simulink model "prct_model_IMV"  (R2018a)
settings: Solver=FixedStepDiscrete  StartTime=0.0  StopTime=3.2  FixedStep=0.01  RelTol=1e-3
model workspace (MAT data in the model file):
  IMV_Time = Simulink.Signal
  IMV_Time.DataType = 'single'
  IMV_Time.Dimensions = -1
  IMV_Time.DimensionsMode = 'auto'
  IMV_Time.Complexity = 'auto'
  IMV_Time.SampleTime = -1
  IMV_Time.SamplingMode = 'auto'
values from neighbouring files (symbols this model uses):
  Diesel_Viscocity = 875.0    [HPP18_DD.sldd]
  Discharge_Coefficient = 0.7    [HPP18_DD.sldd]
  Divide_Constant = 4.0    [HPP18_DD.sldd]
  meterToliter = 1000.0    [HPP18_DD.sldd]
  Orifices_Dia = 0.0035    [HPP18_DD.sldd]
  Pressure_UnitConversion = 200000.0    [HPP18_DD.sldd]
  Time_ScalingFactor = 1000.0    [HPP18_DD.sldd]
undefined symbols (not defined in the file or in its folder): sigbuilder_block
libraries: simulink x2
settings Model: DataDictionary=Pract_IMV.sldd  Creator=Sohan  LastModifiedBy=Sohan
settings OptimizationCC: BlockReduction=off  DefaultParameterBehavior=Inlined  UseDivisionForNetSlopeComputation=on  EnhancedBackFolding=on  PassReuseOutputArgsAs=Individual arguments  EfficientFloat2IntCast=on  LifeSpan=inf  OptimizeBlockOrder=speed  DifferentSizesBufferReuse=on  OptimizationCustomize=off
settings DebuggingCC: SignalInfNanChecking=error  SignalRangeChecking=error  ReadBeforeWriteMsg=EnableAllAsError  WriteAfterWriteMsg=EnableAllAsError  WriteAfterReadMsg=EnableAllAsError  AlgebraicLoopMsg=error  ArtificialAlgebraicLoopMsg=error  SaveWithDisabledLinksMsg=error  SaveWithParameterizedLinksMsg=error  BlockPriorityViolationMsg=error  SolverPrmCheckMsg=error  InheritedTsInSrcMsg=error  SigSpecEnsureSampleTimeMsg=error  CheckMatrixSingularityMsg=error  IntegerOverflowMsg=error  ParameterUnderflowMsg=error  ParameterPrecisionLossMsg=error  ParameterTunabilityLossMsg=error  UnderSpecifiedDataTypeMsg=error  UnnecessaryDatatypeConvMsg=warning  VectorMatrixConversionMsg=error  SignalLabelMismatchMsg=error  UnconnectedInputMsg=error  UnconnectedOutputMsg=error  UnconnectedLineMsg=error  SFcnCompatibilityMsg=error  UniqueDataStoreMsg=warning  BusObjectLabelMismatch=error  RootOutportRequireBusObject=error  AssertControl=DisableAll  ModelReferenceIOMsg=error  ModelReferenceIOMismatchMessage=error  UnknownTsInhSupMsg=error  ModelReferenceDataLoggingMessage=error  StateNameClashWarn=warning  StrictBusMsg=ErrorOnBusTreatedAsVector  SFInvalidInputDataAccessInChartInitDiag=error  SFTransitionOutsideNaturalParentDiag=error  SFUnreachableExecutionPathDiag=error
settings SFSimCC: MATLABDynamicMemAlloc=off
settings RTWCC: SystemTargetFile=ert.tlc  TemplateMakefile=ert_default_tmf  GenerateReport=on  IncludeHyperlinkInReport=on  LaunchReport=on  GenerateTraceInfo=on  GenerateTraceReport=on  GenerateTraceReportSl=on  GenerateTraceReportSf=on  GenerateTraceReportEml=on
settings CodeAppCC: ForceParamTrailComments=on  IgnoreCustomStorageClasses=off  OperatorAnnotations=on  SimulinkDataObjDesc=on  SFDataObjDesc=on  MangleLength=4  InsertBlockDesc=on  ReqsInCode=on
settings ERTTargetCC: TargetLangStandard=C99 (ISO)  UtilityFuncGeneration=Shared location  GenerateSampleERTMain=on  IncludeMdlTerminateFcn=off  SuppressErrorStatus=on  SupportAbsoluteTime=off  SupportNonFinite=off  ParenthesesLevel=Maximum  CastingMode=Standards  GenerateSharedConstants=off  InlinedParameterPlacement=NonHierarchical  ERTCustomFileTemplate=example_file_process.tlc  PreserveExpressionOrder=on  PreserveIfCondition=on  EnableSignedLeftShifts=off  EnableSignedRightShifts=off
settings ConfigComp: CovEnable=on  RecordCoverage=on  CovMetricSettings=dcmwe  CovModelRefEnable=on  DVMaxProcessTime=333  DVModelCoverageObjectives=MCDC  DVTestSuiteOptimization=CombinedObjectives (Nonlinear Extended)  DVDetectDeadLogic=on  DVDetectFloatOverflow=off  DVSaveReport=on

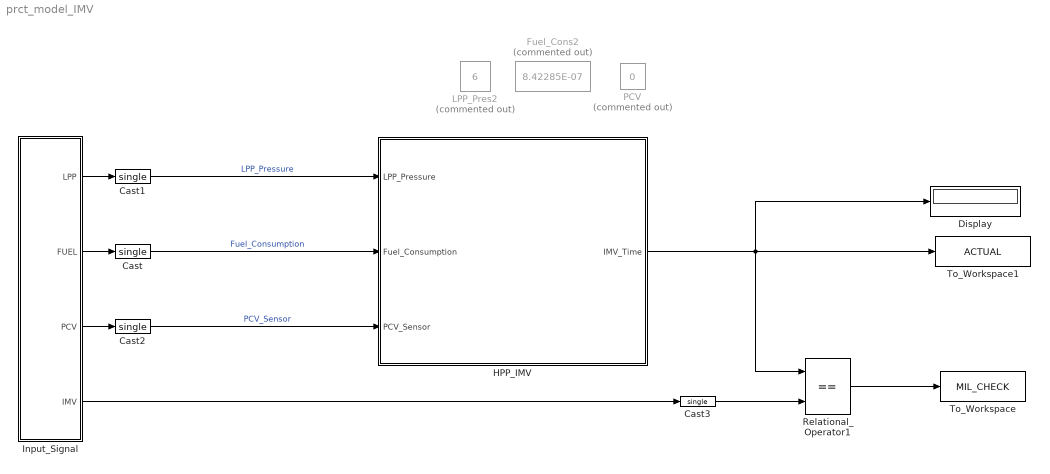
== system prct_model_IMV ==
  Cast{,1..3} (4 alike) : DataTypeConversion  OutDataTypeStr=single
  Display : Display
  Fuel_Cons2 : Constant  Commented=on  Value=8.42285E-07
  HPP_IMV : Subsystem  TreatAsAtomicUnit=on
  Input_Signal : Subsystem  Tag=STV Subsys  LoadFcn=sigbuilder_block('load');  StartFcn=sigbuilder_block('start');  StopFcn=sigbuilder_block('stop');  ClipboardFcn=sigbuilder_block('clipboard');  mask(Sigbuilder block){tuvar=[0:10]}
      mask help: Simulink:masks:SigbuilderBlock_MD
      mask init:
      | if ~strcmp(get_param(bdroot(gcbh),'SimulationStatus'),'stopped') tuvar = sigbuilder_block('maskInit'); end
      settings: CopyFcn=sigbuilder_block('copy');  DeleteFcn=sigbuilder_block('delete');  ModelCloseFcn=sigbuilder_block('modelClose');  PreSaveFcn=sigbuilder_block('preSave');  PauseFcn=sigbuilder_block('pause');  ContinueFcn=sigbuilder_block('continue');  NameChangeFcn=sigbuilder_block('namechange');  OpenFcn=sigbuilder_block('open',[433.2 159.6 550.8 400.2 ]);  CloseFcn=sigbuilder_block('close');
      mask Display: plot(0, 0, 100, 100,[2, 2, 32, 32, 2], [68, 8, 8, 68, 68],[32, 2], [38, 38], [32, 19, 2],[53, 60, 44], [32, 17, 17, 2],[16, 16, 31, 31]);txt = getActiveGroup(gcbh);text(2, 100, txt,'verticalAlignment', 'top');
  LPP_Pres2 : Constant  Commented=on  Value=6  OutDataTypeStr=single
  PCV : Constant  Commented=on  Value=0  OutDataTypeStr=single
  Relational_Operator1 : RelationalOperator  Operator===  OutDataTypeStr=boolean
  To_Workspace : ToWorkspace  VariableName=MIL_CHECK  SaveFormat=Timeseries  SampleTime=-1
  To_Workspace1 : ToWorkspace  VariableName=ACTUAL  SaveFormat=Timeseries  SampleTime=-1
  wires:
  Input_Signal/1(LPP) -> Cast1/1
  Relational_Operator1/1 -> To_Workspace/1
  HPP_IMV/1(IMV_Time) -> To_Workspace1/1, Relational_Operator1/1, Display/1
  Input_Signal/2(FUEL) -> Cast/1
  Cast3/1 -> Relational_Operator1/2
  Cast/1 -> HPP_IMV/2(Fuel_Consumption)  "Fuel_Consumption"
  Input_Signal/4(IMV) -> Cast3/1
  Cast1/1 -> HPP_IMV/1(LPP_Pressure)  "LPP_Pressure"
  Cast2/1 -> HPP_IMV/3(PCV_Sensor)  "PCV_Sensor"
  Input_Signal/3(PCV) -> Cast2/1

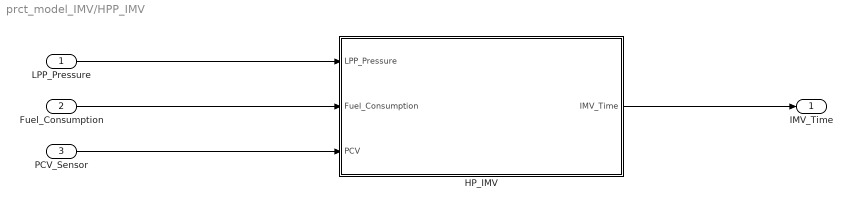
== system prct_model_IMV/HPP_IMV ==
  LPP_Pressure : Inport
  Fuel_Consumption : Inport  Port=2
  PCV_Sensor : Inport  Port=3
  HP_IMV : Subsystem  TreatAsAtomicUnit=on
  IMV_Time : Outport
  wires:
  HP_IMV/1(IMV_Time) -> IMV_Time/1
  Fuel_Consumption/1 -> HP_IMV/2(Fuel_Consumption)
  LPP_Pressure/1 -> HP_IMV/1(LPP_Pressure)
  PCV_Sensor/1 -> HP_IMV/3(PCV)

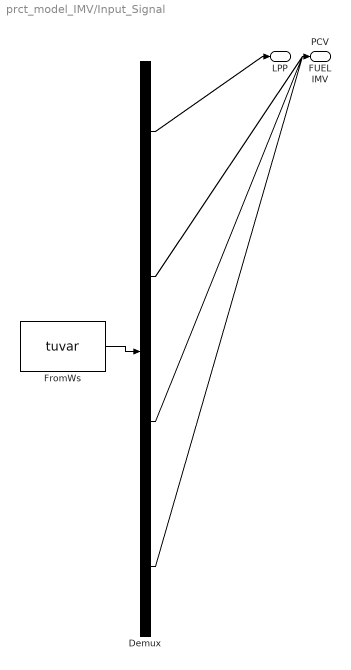
== system prct_model_IMV/Input_Signal ==
  Demux : Demux  Tag=STV Demux
  FromWs : FromWorkspace  Tag=STV FromWs  VariableName=tuvar  SampleTime=0
      SigBuilderData=|
      | common.afterFinalStr = 'Extrapolate'
      | common.sampleTime = 0
      | dataSet.timeRange = [0 3.2]
      | dataSet.name = 'Sheet3'
      | sbobj.Name = 'Signal Builder'
      | sbobj.Groups.Name = 'Sheet3'
      | sbobj.Groups.Signals(1).Name = 'LPP'
      | sbobj.Groups.Signals(1).XData = [0 0.01 0.02 0.03 0.04 0.05 0.06 0.07 0.08 0.09 0.1 0.11 0.12 0.13 0.14 0.15 0.16 0.17 0.18 0.19 0.2 0.21 0.22 0.23 0.24 0.25 0.26 0.27 0.28 0.29 0.3 0.31 0.32 0.33 0.34 0.35 0.36 0.37 0.38 0.39 0.4 0.41 0.42 0.43 0.44 0.45 0.46 0.47 0.48 0.49 0.5 0.51 0.52 0.53 0.54 0.55 0.56 0.57 0.58 0.59 0.6 0.61 0.62 0.63 0.64 0.65 0.66 0.67 0.68 0.69 0.7 0.71 0.72 0.73 0.74 0.75 0.76 0.77 0.78 0.79 0.8 0.81 0.82 0.83 0.84 0.85 0.86 0.87 0.88 0.89 0.9 0.91 0.92 0.93 0.94 0.95 0.96 0.97 0.98 0.99 1 1.01 1.02 1.03 1.04 1.05 1.06 1.07 1.08 1.09 1.1 1.11 1.12 1.13 1.14 1.15 1.16 1.17 1.18 1.19 1.2 1.21 1.22 1.23 1.24 1.25 1.26 1.27 1.28 1.29 1.3 1.31 1.32 1.33 1.34 1.35 1.36 1.37 1.38 1.39 1.4 1.41 1.42 1.43 1.44 1.45 1.46 1.47 1.48 1.49 1.5 1.51 1.52 1.53 1.54 1.55 1.56 1.57 1.58 1.59 1.6 1.61 1.62 1.63 1.64 1.65 1.66 1.67 1.68 1.69 1.7 1.71 1.72 1.73 1.74 1.75 1.76 1.77 1.78 1.79 1.8 1.81 1.82 1.83 1.84 1.85 1.86 1.87 1.88 1.89 1.9 1.91 1.92 1.93 1.94 1.95 1.96 1.97 1.98 1.99 2 2.01 2.02 2.03 2.04 2.05 2.06 2.07 2.08 2.09 2.1 2.11 2.12 2.13 2.14 2.15 2.16 2.17 2.18 2.19 2.2 2.21 2.22 2.23 2.24 2.25 2.26 2.27 2.28 2.29 2.3 2.31 2.32 2.33 2.34 2.35 2.36 2.37 2.38 2.39 2.4 2.41 2.42 2.43 2.44 2.45 2.46 2.47 2.48 2.49 2.5 2.51 2.52 2.53 2.54 2.55 2.56 2.57 2.58 2.59 2.6 2.61 2.62 2.63 2.64 2.65 2.66 2.67 2.68 2.69 2.7 2.71 2.72 2.73 2.74 2.75 2.76 2.77 2.78 2.79 2.8 2.81 2.82 2.83 2.84 2.85 2.86 2.87 2.88 2.89 2.9 2.91 2.92 2.93 2.94 2.95 2.96 2.97 2.98 2.99 3 3.01 3.02 3.03 3.04 3.05 3.06 3.07 3.08 3.09 3.1 3.11 3.12 3.13 3.14 3.15 3.16 3.17 3.18 3.19 3.2]
      | sbobj.Groups.Signals(1).YData = [-1 6 6 6 6 6 6 6 6 6 6 6 6 6 6 6 6 6 6 6 6 6 6 6 6 6 6 6 6 6 6 6 6 6 6 6 6 6 6 6 6 6 6 6 6 6 6 6 6 6 6 6 6 6 6 6 6 6 6 6 6 6 6 6 6 6 6 6 6 6 6 6 6 6 6 6 6 6 6 6 6 6 6 6 6 6 6 6 6 6 6 6 6 6 6 6 6 6 6 6 6 6 6 6 6 6 6 6 6 6 6 6 6 6 6 6 6 6 6 6 6 6 6 6 6 6 6 6 6 6 6 6 6 6 6 6 6 6 6 6 6 6 6 6 6 6 6 6 6 6 6 6 6 6 6 6 6 6 6 6 6 6 6 6 6 6 6 6 6 6 6 6 6 6 6 6 6 6 6 6 6 6 6 6 6 6 6 6 6 6 6 6 6 6 6 6 6 6 6 6 6 6 6 6 6 6 6 6 6 6 6 6 6 6 6 6 6 6 6 6 6 6 6 6 6 6 6 6 6 6 6 6 6 6 6 6 6 6 6 6 6 6 6 6 6 6 6 6 6 6 6 6 6 6 6 6 6 6 6 6 6 6 6 6 6 6 6 6 6 6 6 6 6 6 6 6 6 6 6 6 6 6 6 6 6 6 6 6 6 6 6 6 6 6 6 6 6 6 6 6 6 6 6 6 6 6 6 6 6 6 6 6 6 6 6 6 6 6 6 6 6]
      | sbobj.Groups.Signals(2).Name = 'FUEL'
      | sbobj.Groups.Signals(2).XData = [0 0.01 0.02 0.03 0.04 0.05 0.06 0.07 0.08 0.09 0.1 0.11 0.12 0.13 0.14 0.15 0.16 0.17 0.18 0.19 0.2 0.21 0.22 0.23 0.24 0.25 0.26 0.27 0.28 0.29 0.3 0.31 0.32 0.33 0.34 0.35 0.36 0.37 0.38 0.39 0.4 0.41 0.42 0.43 0.44 0.45 0.46 0.47 0.48 0.49 0.5 0.51 0.52 0.53 0.54 0.55 0.56 0.57 0.58 0.59 0.6 0.61 0.62 0.63 0.64 0.65 0.66 0.67 0.68 0.69 0.7 0.71 0.72 0.73 0.74 0.75 0.76 0.77 0.78 0.79 0.8 0.81 0.82 0.83 0.84 0.85 0.86 0.87 0.88 0.89 0.9 0.91 0.92 0.93 0.94 0.95 0.96 0.97 0.98 0.99 1 1.01 1.02 1.03 1.04 1.05 1.06 1.07 1.08 1.09 1.1 1.11 1.12 1.13 1.14 1.15 1.16 1.17 1.18 1.19 1.2 1.21 1.22 1.23 1.24 1.25 1.26 1.27 1.28 1.29 1.3 1.31 1.32 1.33 1.34 1.35 1.36 1.37 1.38 1.39 1.4 1.41 1.42 1.43 1.44 1.45 1.46 1.47 1.48 1.49 1.5 1.51 1.52 1.53 1.54 1.55 1.56 1.57 1.58 1.59 1.6 1.61 1.62 1.63 1.64 1.65 1.66 1.67 1.68 1.69 1.7 1.71 1.72 1.73 1.74 1.75 1.76 1.77 1.78 1.79 1.8 1.81 1.82 1.83 1.84 1.85 1.86 1.87 1.88 1.89 1.9 1.91 1.92 1.93 1.94 1.95 1.96 1.97 1.98 1.99 2 2.01 2.02 2.03 2.04 2.05 2.06 2.07 2.08 2.09 2.1 2.11 2.12 2.13 2.14 2.15 2.16 2.17 2.18 2.19 2.2 2.21 2.22 2.23 2.24 2.25 2.26 2.27 2.28 2.29 2.3 2.31 2.32 2.33 2.34 2.35 2.36 2.37 2.38 2.39 2.4 2.41 2.42 2.43 2.44 2.45 2.46 2.47 2.48 2.49 2.5 2.51 2.52 2.53 2.54 2.55 2.56 2.57 2.58 2.59 2.6 2.61 2.62 2.63 2.64 2.65 2.66 2.67 2.68 2.69 2.7 2.71 2.72 2.73 2.74 2.75 2.76 2.77 2.78 2.79 2.8 2.81 2.82 2.83 2.84 2.85 2.86 2.87 2.88 2.89 2.9 2.91 2.92 2.93 2.94 2.95 2.96 2.97 2.98 2.99 3 3.01 3.02 3.03 3.04 3.05 3.06 3.07 3.08 3.09 3.1 3.11 3.12 3.13 3.14 3.15 3.16 3.17 3.18 3.19 3.2]
      | sbobj.Groups.Signals(2).YData = [0 8.4228515625e-07 1.6845703125e-06 2.52685546875e-06 3.369140625e-06 4.21142578125e-06 5.0537109375e-06 5.89599609375e-06 6.73828125e-06 7.58056640625e-06 8.4228515625e-06 9.26513671875e-06 ... (321 elements, 1x321)]
      | sbobj.Groups.Signals(3).Name = 'PCV'
      | sbobj.Groups.Signals(3).XData = [0 0.01 0.02 0.03 0.04 0.05 0.06 0.07 0.08 0.09 0.1 0.11 0.12 0.13 0.14 0.15 0.16 0.17 0.18 0.19 0.2 0.21 0.22 0.23 0.24 0.25 0.26 0.27 0.28 0.29 0.3 0.31 0.32 0.33 0.34 0.35 0.36 0.37 0.38 0.39 0.4 0.41 0.42 0.43 0.44 0.45 0.46 0.47 0.48 0.49 0.5 0.51 0.52 0.53 0.54 0.55 0.56 0.57 0.58 0.59 0.6 0.61 0.62 0.63 0.64 0.65 0.66 0.67 0.68 0.69 0.7 0.71 0.72 0.73 0.74 0.75 0.76 0.77 0.78 0.79 0.8 0.81 0.82 0.83 0.84 0.85 0.86 0.87 0.88 0.89 0.9 0.91 0.92 0.93 0.94 0.95 0.96 0.97 0.98 0.99 1 1.01 1.02 1.03 1.04 1.05 1.06 1.07 1.08 1.09 1.1 1.11 1.12 1.13 1.14 1.15 1.16 1.17 1.18 1.19 1.2 1.21 1.22 1.23 1.24 1.25 1.26 1.27 1.28 1.29 1.3 1.31 1.32 1.33 1.34 1.35 1.36 1.37 1.38 1.39 1.4 1.41 1.42 1.43 1.44 1.45 1.46 1.47 1.48 1.49 1.5 1.51 1.52 1.53 1.54 1.55 1.56 1.57 1.58 1.59 1.6 1.61 1.62 1.63 1.64 1.65 1.66 1.67 1.68 1.69 1.7 1.71 1.72 1.73 1.74 1.75 1.76 1.77 1.78 1.79 1.8 1.81 1.82 1.83 1.84 1.85 1.86 1.87 1.88 1.89 1.9 1.91 1.92 1.93 1.94 1.95 1.96 1.97 1.98 1.99 2 2.01 2.02 2.03 2.04 2.05 2.06 2.07 2.08 2.09 2.1 2.11 2.12 2.13 2.14 2.15 2.16 2.17 2.18 2.19 2.2 2.21 2.22 2.23 2.24 2.25 2.26 2.27 2.28 2.29 2.3 2.31 2.32 2.33 2.34 2.35 2.36 2.37 2.38 2.39 2.4 2.41 2.42 2.43 2.44 2.45 2.46 2.47 2.48 2.49 2.5 2.51 2.52 2.53 2.54 2.55 2.56 2.57 2.58 2.59 2.6 2.61 2.62 2.63 2.64 2.65 2.66 2.67 2.68 2.69 2.7 2.71 2.72 2.73 2.74 2.75 2.76 2.77 2.78 2.79 2.8 2.81 2.82 2.83 2.84 2.85 2.86 2.87 2.88 2.89 2.9 2.91 2.92 2.93 2.94 2.95 2.96 2.97 2.98 2.99 3 3.01 3.02 3.03 3.04 3.05 3.06 3.07 3.08 3.09 3.1 3.11 3.12 3.13 3.14 3.15 3.16 3.17 3.18 3.19 3.2]
      | sbobj.Groups.Signals(3).YData = [0 0 0 0 0 0 0 0 0 0 0 0 0 0 0 0 0 0 0 0 0 0 0 0 0 0 0 0 0 0 0 0 0 0 0 0 0 0 0 0 0 0 0 0 0 0 1 1 1 1 1 1 1 1 1 1 1 1 1 1 1 1 1 1 1 1 1 1 1 1 1 1 1 1 1 1 1 1 1 1 1 1 1 1 1 1 1 1 1 1 1 1 1 1 1 1 1 1 1 1 1 1 1 1 1 1 1 1 1 1 1 1 1 1 1 1 1 1 1 1 1 1 1 1 1 1 1 1 1 1 1 1 1 1 1 1 1 1 1 1 1 1 1 1 1 1 1 1 1 1 1 1 1 1 1 1 1 1 1 1 1 1 1 1 1 1 1 1 1 1 1 1 1 1 1 1 1 1 1 1 1 1 1 1 1 1 1 1 1 1 1 1 1 1 0 0 0 0 0 0 0 0 0 0 0 0 0 0 0 0 0 0 0 0 0 0 0 0 0 0 0 0 0 0 0 0 0 0 0 0 0 0 0 0 0 0 0 0 0 0 0 0 0 0 0 0 0 0 0 0 0 0 0 0 0 0 0 0 0 0 0 0 0 0 0 0 0 0 0 0 0 0 0 0 0 0 0 0 0 0 0 0 0 0 0 0 0 0 0 0 0 0 0 0 0 0 0 0 0 0 0 0 0 0 0 0 0 0 0 0 0 0 0 0 0 0 0 0 0 0 0]
      | sbobj.Groups.Signals(4).Name = 'IMV'
      | sbobj.Groups.Signals(4).XData = [0 0.01 0.02 0.03 0.04 0.05 0.06 0.07 0.08 0.09 0.1 0.11 0.12 0.13 0.14 0.15 0.16 0.17 0.18 0.19 0.2 0.21 0.22 0.23 0.24 0.25 0.26 0.27 0.28 0.29 0.3 0.31 0.32 0.33 0.34 0.35 0.36 0.37 0.38 0.39 0.4 0.41 0.42 0.43 0.44 0.45 0.46 0.47 0.48 0.49 0.5 0.51 0.52 0.53 0.54 0.55 0.56 0.57 0.58 0.59 0.6 0.61 0.62 0.63 0.64 0.65 0.66 0.67 0.68 0.69 0.7 0.71 0.72 0.73 0.74 0.75 0.76 0.77 0.78 0.79 0.8 0.81 0.82 0.83 0.84 0.85 0.86 0.87 0.88 0.89 0.9 0.91 0.92 0.93 0.94 0.95 0.96 0.97 0.98 0.99 1 1.01 1.02 1.03 1.04 1.05 1.06 1.07 1.08 1.09 1.1 1.11 1.12 1.13 1.14 1.15 1.16 1.17 1.18 1.19 1.2 1.21 1.22 1.23 1.24 1.25 1.26 1.27 1.28 1.29 1.3 1.31 1.32 1.33 1.34 1.35 1.36 1.37 1.38 1.39 1.4 1.41 1.42 1.43 1.44 1.45 1.46 1.47 1.48 1.49 1.5 1.51 1.52 1.53 1.54 1.55 1.56 1.57 1.58 1.59 1.6 1.61 1.62 1.63 1.64 1.65 1.66 1.67 1.68 1.69 1.7 1.71 1.72 1.73 1.74 1.75 1.76 1.77 1.78 1.79 1.8 1.81 1.82 1.83 1.84 1.85 1.86 1.87 1.88 1.89 1.9 1.91 1.92 1.93 1.94 1.95 1.96 1.97 1.98 1.99 2 2.01 2.02 2.03 2.04 2.05 2.06 2.07 2.08 2.09 2.1 2.11 2.12 2.13 2.14 2.15 2.16 2.17 2.18 2.19 2.2 2.21 2.22 2.23 2.24 2.25 2.26 2.27 2.28 2.29 2.3 2.31 2.32 2.33 2.34 2.35 2.36 2.37 2.38 2.39 2.4 2.41 2.42 2.43 2.44 2.45 2.46 2.47 2.48 2.49 2.5 2.51 2.52 2.53 2.54 2.55 2.56 2.57 2.58 2.59 2.6 2.61 2.62 2.63 2.64 2.65 2.66 2.67 2.68 2.69 2.7 2.71 2.72 2.73 2.74 2.75 2.76 2.77 2.78 2.79 2.8 2.81 2.82 2.83 2.84 2.85 2.86 2.87 2.88 2.89 2.9 2.91 2.92 2.93 2.94 2.95 2.96 2.97 2.98 2.99 3 3.01 3.02 3.03 3.04 3.05 3.06 3.07 3.08 3.09 3.1 3.11 3.12 3.13 3.14 3.15 3.16 3.17 3.18 3.19 3.2]
      | sbobj.Groups.Signals(4).YData = [0 0.00337884466688 0.00675768933377 0.0101365340006 0.0135153786675 0.0168942233344 0.0202730680013 0.0236519126682 0.0270307573351 0.0304096020019 0.0337884466688 0.0371672913357 ... (321 elements, 1x321)]
      | sbobj.Groups.TimeRange = [0 3.2]
  LPP : Outport  Tag=STV Outport
  FUEL : Outport  Tag=STV Outport  Port=2
  PCV : Outport  Tag=STV Outport  Port=3
  IMV : Outport  Tag=STV Outport  Port=4
  wires:
  Demux/3 -> PCV/1
  FromWs/1 -> Demux/1
  Demux/1 -> LPP/1
  Demux/2 -> FUEL/1
  Demux/4 -> IMV/1

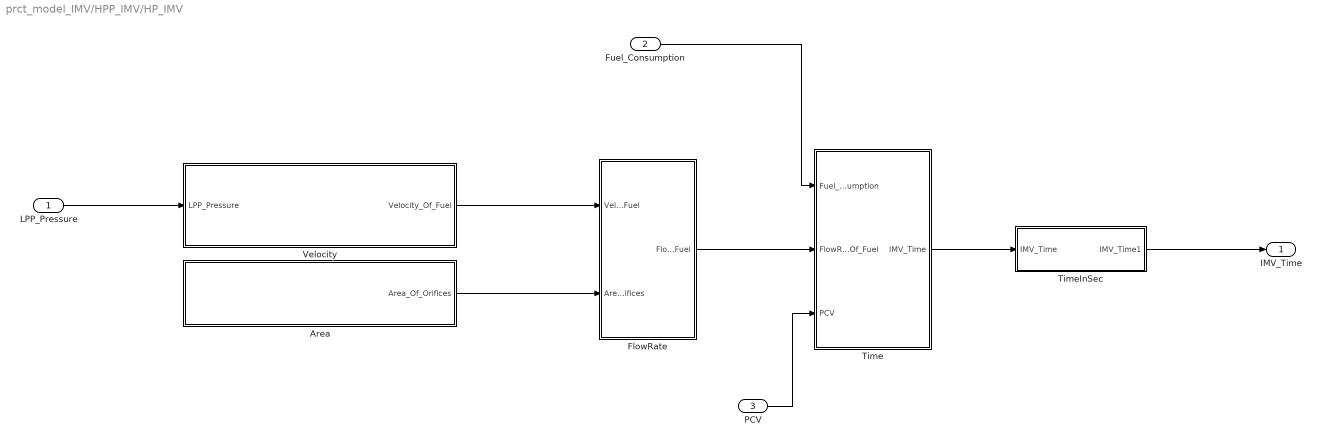
== system prct_model_IMV/HPP_IMV/HP_IMV ==
  LPP_Pressure : Inport
  Fuel_Consumption : Inport  Port=2
  PCV : Inport  Port=3
  Area : Subsystem
  FlowRate : Subsystem
  Time : Subsystem
  TimeInSec : Subsystem
  Velocity : Subsystem
  IMV_Time : Outport
  wires:
  Area/1(Area_Of_Orifices) -> FlowRate/2(Area_Of_Orifices)
  FlowRate/1(FlowRate_Of_Fuel) -> Time/2(FlowRate_Of_Fuel)
  Velocity/1(Velocity_Of_Fuel) -> FlowRate/1(Velocity_Of_Fuel)
  Fuel_Consumption/1 -> Time/1(Fuel_Consumption)
  Time/1(IMV_Time) -> TimeInSec/1(IMV_Time)
  TimeInSec/1(IMV_Time1) -> IMV_Time/1
  LPP_Pressure/1 -> Velocity/1(LPP_Pressure)
  PCV/1 -> Time/3(PCV)

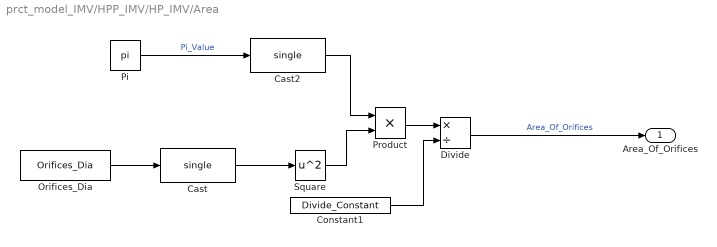
== system prct_model_IMV/HPP_IMV/HP_IMV/Area ==
  Cast : DataTypeConversion  OutDataTypeStr=single
  Cast2 : DataTypeConversion  OutDataTypeStr=single
  Constant1 : Constant  Value=Divide_Constant  OutDataTypeStr=single
  Divide : Product  Inputs=*/
  Orifices_Dia : Constant  Value=Orifices_Dia  OutDataTypeStr=double
  Pi : Constant  Value=pi  OutDataTypeStr=double
  Product : Product
  Square : Math  Operator=square  SaturateOnIntegerOverflow=on
  Area_Of_Orifices : Outport
  wires:
  Orifices_Dia/1 -> Cast/1
  Square/1 -> Product/2
  Product/1 -> Divide/1
  Constant1/1 -> Divide/2
  Divide/1 -> Area_Of_Orifices/1  "Area_Of_Orifices"
  Cast2/1 -> Product/1
  Pi/1 -> Cast2/1  "Pi_Value"
  Cast/1 -> Square/1

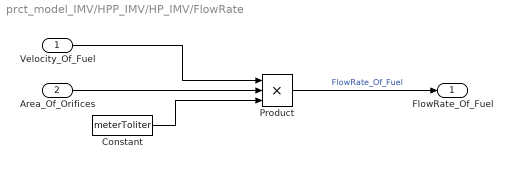
== system prct_model_IMV/HPP_IMV/HP_IMV/FlowRate ==
  Velocity_Of_Fuel : Inport
  Area_Of_Orifices : Inport  Port=2
  Constant : Constant  Value=meterToliter  OutDataTypeStr=single
  Product : Product  Inputs=3
  FlowRate_Of_Fuel : Outport
  wires:
  Area_Of_Orifices/1 -> Product/2
  Velocity_Of_Fuel/1 -> Product/1
  Constant/1 -> Product/3
  Product/1 -> FlowRate_Of_Fuel/1  "FlowRate_Of_Fuel"

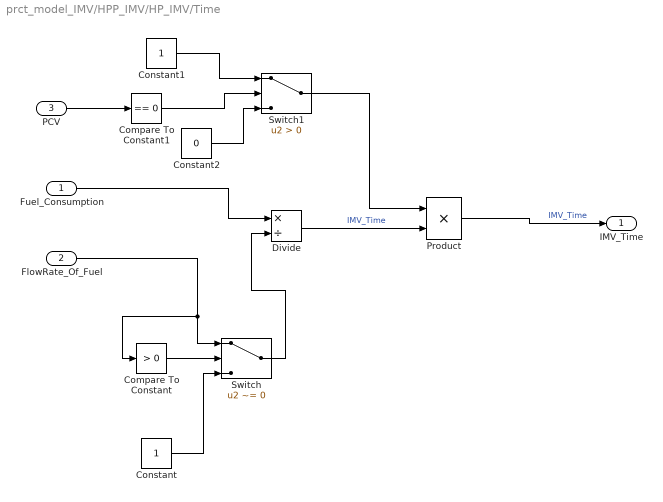
== system prct_model_IMV/HPP_IMV/HP_IMV/Time ==
  Fuel_Consumption : Inport
  FlowRate_Of_Fuel : Inport  Port=2
  PCV : Inport  Port=3
  Compare To Constant : simulink/Logic and Bit Operations/Compare To Constant  relop=>  const=0  OutDataTypeStr=boolean
  Compare To Constant1 : simulink/Logic and Bit Operations/Compare To Constant  relop===  const=0  OutDataTypeStr=boolean
  Constant : Constant  OutDataTypeStr=single
  Constant1 : Constant  OutDataTypeStr=single
  Constant2 : Constant  Value=0  OutDataTypeStr=single
  Divide : Product  Inputs=*/
  Product : Product
  Switch : Switch  Criteria=u2 ~= 0
  Switch1 : Switch  Criteria=u2 > Threshold
  IMV_Time : Outport
  wires:
  Fuel_Consumption/1 -> Divide/1
  FlowRate_Of_Fuel/1 -> Compare To Constant/1, Switch/1
  Product/1 -> IMV_Time/1  "IMV_Time"
  Divide/1 -> Product/2  "IMV_Time"
  Switch1/1 -> Product/1
  PCV/1 -> Compare To Constant1/1
  Compare To Constant/1 -> Switch/2
  Constant/1 -> Switch/3
  Switch/1 -> Divide/2
  Compare To Constant1/1 -> Switch1/2
  Constant1/1 -> Switch1/1
  Constant2/1 -> Switch1/3

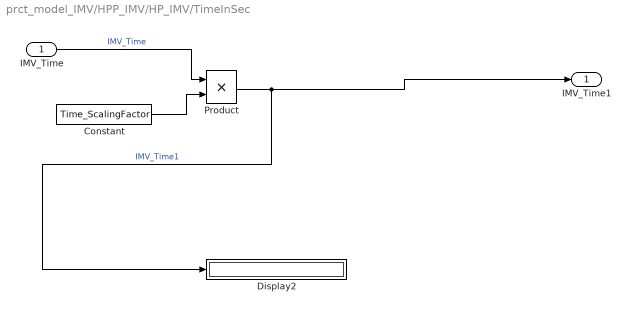
== system prct_model_IMV/HPP_IMV/HP_IMV/TimeInSec ==
  IMV_Time : Inport
  Constant : Constant  Value=Time_ScalingFactor  OutDataTypeStr=single
  Display2 : Display
  Product : Product  RndMeth=Ceiling
  IMV_Time1 : Outport
  wires:
  IMV_Time/1 -> Product/1  "IMV_Time"
  Product/1 -> Display2/1, IMV_Time1/1  "IMV_Time1"
  Constant/1 -> Product/2

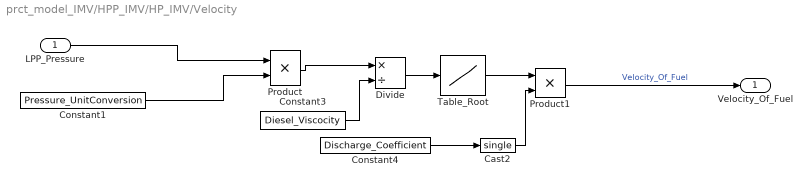
== system prct_model_IMV/HPP_IMV/HP_IMV/Velocity ==
  LPP_Pressure : Inport
  Cast2 : DataTypeConversion  OutDataTypeStr=single
  Constant1 : Constant  Value=Pressure_UnitConversion  OutDataTypeStr=single
  Constant3 : Constant  Value=Diesel_Viscocity  OutDataTypeStr=single
  Constant4 : Constant  Value=Discharge_Coefficient
  Divide : Product  Inputs=*/
  Product : Product
  Product1 : Product
  "Table_Root " : Lookup_n-D  NumberOfTableDimensions=1  BreakpointsForDimension1=|  Table=|  InternalRulePriority=Speed  InputSameDT=on
      BreakpointsForDimension1=|
      | [
      | 
      | 0
      | 1
      | 4
      | 9
      | 16
      | 25
      | 36
      | 49
      | 64
      | 81
      | 100
      | 121
      | 144
      | 169
      | 196
      | 225
      | 256
      | 289
      | 324
      | 361
      | 400
      | 441
      | 484
      | 529
      | 576
      | 625
      | 676
      | 729
      | 784
      | 841
      | 900
      | 961
      | 1024
      | 1089
      | 1156
      | 1225
      | 1296
      | 1369
      | 1444
      | 1521
      | 1600
      | 1681
      | 1764
      | 1849
      | 1936
      | 2025
      | 2116
      | 2209
      | 2304
      | 2401
      | 2500
      |  
      | ]
      Table=|
      | [
      | 
      | 0
      | 1
      | 2
      | 3
      | 4
      | 5
      | 6
      | 7
      | 8
      | 9
      | 10
      | 11
      | 12
      | 13
      | 14
      | 15
      | 16
      | 17
      | 18
      | 19
      | 20
      | 21
      | 22
      | 23
      | 24
      | 25
      | 26
      | 27
      | 28
      | 29
      | 30
      | 31
      | 32
      | 33
      | 34
      | 35
      | 36
      | 37
      | 38
      | 39
      | 40
      | 41
      | 42
      | 43
      | 44
      | 45
      | 46
      | 47
      | 48
      | 49
      | 50
      | ]
  Velocity_Of_Fuel : Outport
  wires:
  LPP_Pressure/1 -> Product/1
  Constant3/1 -> Divide/2
  Constant1/1 -> Product/2
  Product/1 -> Divide/1
  Constant4/1 -> Cast2/1
  "Table_Root "/1 -> Product1/1
  Product1/1 -> Velocity_Of_Fuel/1  "Velocity_Of_Fuel"
  Divide/1 -> "Table_Root "/1
  Cast2/1 -> Product1/2
